simulink model "TestIMU"  (R2016b)
settings: Solver=VariableStepAuto  StartTime=0.0  StopTime=10.0  RelTol=1e-3
model workspace (MATLAB code in the model file):
  | wsHandle = get_param(bdroot, 'modelWorkspace');
  | wsHandle.assignin('sens', AC.Sensors.IMU);
libraries: Sensors_Lib x4
settings Model: Creator=rega0051  LastModifiedBy=rega0051

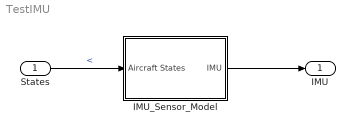
== system TestIMU ==
  "States " : Inport  OutDataTypeStr=Bus: States
  IMU_Sensor_Model : Subsystem  Variant=on  VariantControl=VarIMU_Pass
  " IMU" : Outport  OutDataTypeStr=Bus: IMU
  wires:
  "States "/1 -> IMU_Sensor_Model/1("Aircraft States ")  "<"
  IMU_Sensor_Model/1(" IMU") -> " IMU"/1

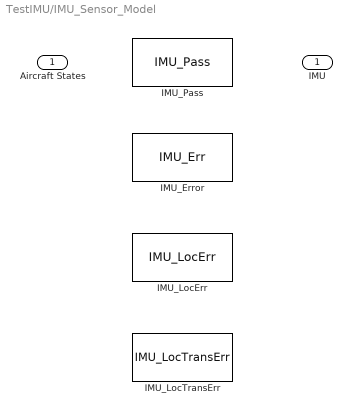
== system TestIMU/IMU_Sensor_Model ==
  "Aircraft States " : Inport
  IMU_Error : Sensors_Lib/IMU Sensor Models/IMU_Err  VariantControl=VarImu_Err
      settings: AttributesFormatString=Variant: %<VariantControl> : %<Variant>
  IMU_LocErr : Sensors_Lib/IMU Sensor Models/IMU_LocErr  VariantControl=VarImu_LocErr
      settings: AttributesFormatString=Variant: %<VariantControl> : %<Variant>
  IMU_LocTransErr : Sensors_Lib/IMU Sensor Models/IMU_LocTransErr  VariantControl=VarImu_LocTransErr
      settings: AttributesFormatString=Variant: %<VariantControl> : %<Variant>
  IMU_Pass : Sensors_Lib/IMU Sensor Models/IMU_Pass  VariantControl=VarImu_Pass
      settings: AttributesFormatString=Variant: %<VariantControl> : %<Variant>
  " IMU" : Outport
